simulink model "test3"  (R2016a)
settings: Solver=VariableStepAuto  StartTime=0.0  StopTime=10.0  RelTol=1e-3
libraries: LibrarySimulinkSAS x2
settings Model: Creator=santd  LastModifiedBy=santd

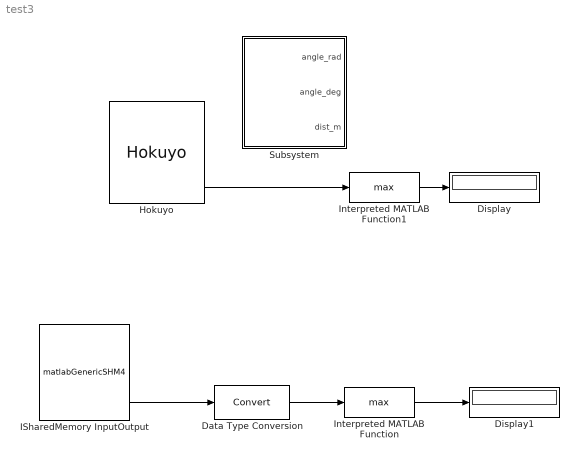
== system test3 ==
  Data Type Conversion : DataTypeConversion
  Display : Display
  Display1 : Display
  Hokuyo : LibrarySimulinkSAS/Hokuyo  SystemSampleTime=-1
  ISharedMemory InputOutput : S-Function  FunctionName=matlabGenericSHM4  Parameters=nameIn,nameOut,vecE,vecS,tipoE,tipoS,ts,trigg,inOff,outOff  SFunctionDeploymentMode=off  EnableBusSupport=off  mask(Generic Share Memory block V2.0){nameIn='none', nameOut='MemoriaHokuyo1_out', vecE=[], vecS=[1 1 1]*683, tipoE=[], tipoS=['f' 'f' 'f'], ts=-1, inOff=0, outOff=0, trigg=off}
      mask prompts: nameIn "Input Shared Memory Name"; nameOut "Output Shared Memory Name"; vecE "Vector of system inputs"; vecS "Vector of system outputs"; tipoE "Data Types Inputs"; tipoS "Data Types Outputs"; ts "Sample Time"; inOff "Input Shared Memory Offset"; outOff "Output Shared Memory Offset"; trigg "Triggered writing"
      mask help:
      | This block allows Simulink communication with external processes through shared memory. It works on Unix and Windows.
      | More information in Help.
      mask Help:
      | Input Shared Memory Name: Name of the memory from which the physical device acquires its inputs.
      | Output Shared Memory Name: Name of the memory in which the physical device writes its output data.
      | Vector of system inputs: array that specify the number of inputs (array dimension) and the inputs size (array values)
      | Vector of system outputs: array that specify the number of outputs (array dimension) and the outputs size (array values)
      | Data types input: char array that specify each input types
      | Data types output: char array that specify each output types
      | Allowed types are:
      | ('f'=float, 'd'=double, 'i'=int32, 'c'=char, 'C'= unsigned char, 'I'=unsigned int)
      | 
      | Triggered writing: If trigger writing is selected, an additional block input is created at the end of inputs. When this input has a value greater than zero the data at the input of the block is written to the device input shared memory, otherwise the data is notwritten.
      | 
      | Example.
      | Suppose the following parameters:
      | Input Shared Memory Name = "devIn_1"
      | Output Shared Memory Name = "devOut_1"
      | Vector of system inputs=[3 2 1]
      | Vector of system outputs=[6 5 7 8]
      | Data types output=['f' 'I' 'c']
      | tipoS=['C' 'i' 'd' 'd']
      | 
      | Two Share Memories are created with names:
      | "devIn_1"(block input)
      | "devOut_1"  (block output)
      | 3 inputs are created:
      |  1° Dimension 3, type "unsigned char"
      |  2° Dimension 2, type "int"
      |  3° Dimension 1, type "char"
      | 4 outputs are created:
      |  1° Dimension 6, type "float"
      |  2° Dimension 5, type "unsigned int"
      |  3° Dimension 7, type "double"
      |  3° Dimension 8, type "double"
      mask Display: image('mem4.png')
  Interpreted MATLAB Function : MATLABFcn  MATLABFcn=max
  Interpreted MATLAB Function1 : MATLABFcn  MATLABFcn=max
  Subsystem : Subsystem
      mask Display:
      | image('hokuyo.jpg')
      | color('red');
      | port_label('output', 1, 'Angle[rad]')
      | port_label('output', 2, 'Angle[deg]')
      | port_label('output', 3, 'Distance[m]')
  wires:
  Hokuyo/3 -> Interpreted MATLAB Function1/1
  ISharedMemory InputOutput/3 -> Data Type Conversion/1
  Interpreted MATLAB Function/1 -> Display1/1
  Interpreted MATLAB Function1/1 -> Display/1
  Data Type Conversion/1 -> Interpreted MATLAB Function/1

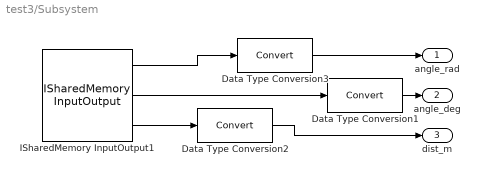
== system test3/Subsystem ==
  Data Type Conversion1 : DataTypeConversion
  Data Type Conversion2 : DataTypeConversion
  Data Type Conversion3 : DataTypeConversion
  ISharedMemory InputOutput1 : LibrarySimulinkSAS/ISharedMemory InputOutput  nameIn='device_input'  nameOut='device_output'  vecE=[]  vecS=[1 1 1]  tipoE=[]  tipoS=['f' 'f' 'f']  ts=-1  trigg=off
  angle_rad : Outport
  angle_deg : Outport  Port=2
  dist_m : Outport  Port=3
  wires:
  ISharedMemory InputOutput1/1 -> Data Type Conversion3/1
  Data Type Conversion1/1 -> angle_deg/1
  ISharedMemory InputOutput1/2 -> Data Type Conversion1/1
  Data Type Conversion3/1 -> angle_rad/1
  ISharedMemory InputOutput1/3 -> Data Type Conversion2/1
  Data Type Conversion2/1 -> dist_m/1
